simulink library "mobileRoboticsLib"  (R2018a)
settings: Solver=VariableStepAuto  StartTime=0.0  StopTime=10.0  RelTol=1e-3
undefined symbols (not defined in the file or in its folder): DiscIntNeverNeededParam, X, Y, Z
libraries: sm_lib x67, nesl_utility x25, $bdroot x11
(part 1 of 4)
settings Model: Creator=scastro  LastModifiedBy=scastro

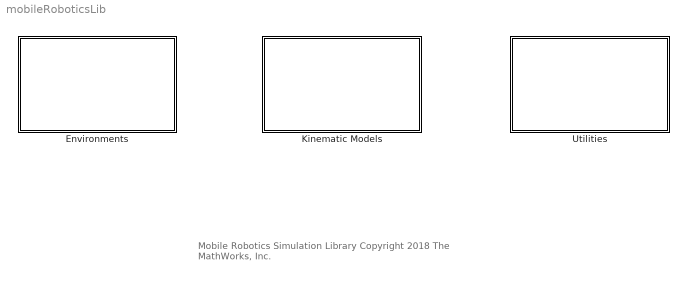
== system mobileRoboticsLib ==
  note: Mobile Robotics Simulation Library
      |
      | Copyright 2018 The MathWorks, Inc.
  Environments : Subsystem
      mask Display: image('environments.PNG');
  Kinematic Models : Subsystem
      mask Display: image('kinematics.PNG')
  Utilities : Subsystem
      mask Display: image('mrsUtils.PNG');

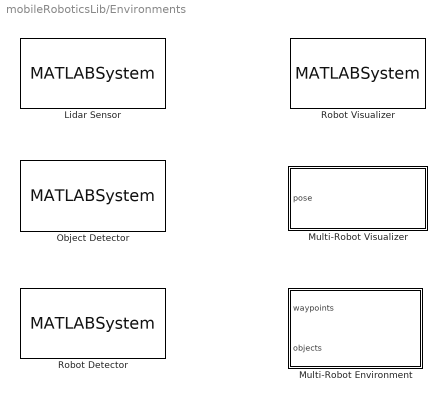
== system mobileRoboticsLib/Environments ==
  Lidar Sensor : MATLABSystem  System=LidarSensor  sensorOffset=[ 0, 0 ]  scanAngles=[ -pi/4, 0, pi/4 ]  maxRange=5  isMultiRobot=off  robotIdx=1
      mask Type: LidarSensor
      mask Display:
      | disp(['Lidar' char(10) 'Sensor']);
      | port_label('input',1,'pose');
      | port_label('output',1,'ranges');
  Multi-Robot Environment : Subsystem  InitFcn=|  TreatAsAtomicUnit=on  mask(Multi-Robot Environment){numRobots=3, mapName=, showWaypoints=on, showObjects=on, showRobotIds=on, plotSensorLines=on}
      | global slMultiRobotEnv;
      | numRobots = str2num(get_param(gcb,'numRobots'));
      | slMultiRobotEnv = MultiRobotEnv(numRobots);
      | slMultiRobotEnv.hasWaypoints = true;
      mask prompts: numRobots "Number of Robots"; mapName "Map Name"; showWaypoints "Accept Waypoints"; showObjects "Accept Objects"; showRobotIds "Show Robot IDs"; plotSensorLines "Plot Sensor Lines"
      mask help:
      | Displays map, waypoint, and object data for a multi-robot simulation.
      |
      | Use "Multi-Robot Visualizer" blocks to display individual robots in this environment.
      mask init:
      | % Configure waypoints port
      | hasWaypointPort = isempty(find_system(gcb,'FollowLinks','on','LookUnderMasks','on','BlockType','Inport','Name','waypoints'));
      | if ~showWaypoints & ~hasWaypointPort
      |     replace_block(gcb,'FollowLinks','on','Name','waypoints','built-in/Ground','noprompt');
      |     hasWaypointPort = false;
      | elseif showWaypoints & hasWaypointPort
      |     replace_block(gcb,'FollowLinks','on','Name','waypoints','built-in/Inport','noprompt'); 
      |     hasWaypointPort = true;
      | end
      | 
      | % Configure objects port
      | hasObjectPort = isempty(find_system(gcb,'FollowLinks','on','LookUnderMasks','on','BlockType','Inport','Name','objects'));
      | if ~showObjects & ~hasObjectPort
      |     replace_block(gcb,'FollowLinks','on','Name','objects','built-in/Ground','noprompt');
      |     hasObjectPort = false;
      | elseif showObjects & hasObjectPort
      |     replace_block(gcb,'FollowLinks','on','Name','objects','built-in/Inport','noprompt');  
      |     hasObjectPort = true;
      | end
      | 
      | % Ensure the waypoints and objects ports are organized correctly
      | if strcmp(get_param([gcb '/waypoints'],'BlockType'),'Inport')
      |     set_param([gcb '/waypoints'],'Port','1');
      | end
      | 
      | 
      | global slMultiRobotEnv
      | if isa(slMultiRobotEnv,'MultiRobotEnv')
      |     release(slMultiRobotEnv) 
      |     slMultiRobotEnv.numRobots = numRobots;
      |     slMultiRobotEnv.mapName = mapName;
      |     slMultiRobotEnv.plotSensorLines = plotSensorLines;
      |     slMultiRobotEnv.showRobotIds = showRobotIds;
      | 
      |     % Show the visualizer
      |     setupVisualization(slMultiRobotEnv);
      | end
      mask Help: web('matlab: edit mrsDocMultiRobotEnv')
      mask Display: fprintf('Multi-Robot\nEnvironment')
  Multi-Robot Visualizer : Subsystem  mask(Multi-Robot Visualizer){idx=1, radius=0, showTraj=on, hasLidar=off, sensorOffset=[0,0], scanAngles=[-pi/4, 0, pi/4], hasObjDetector=off, objDetectorOffset=[0,0], objDetectorAngle=0, objDetectorFOV=pi/3, objDetectorMaxRange=5}
      mask prompts: idx "Robot Index"; radius "Robot Radius [m]"; showTraj "Show Trajectory"; hasLidar "Accept Lidar"; sensorOffset "Lidar sensor offset (x,y) [m]"; scanAngles "Scan angles [rad]"; hasObjDetector "Accept Object Detector"; objDetectorOffset "Object detector offset (x,y) [m]"; objDetectorAngle "Object detector angle [rad]"; objDetectorFOV "Sensor field of view [rad]"; objDetectorMaxRange "Maximum range [m]"
      mask help:
      | Supply the pose and (optionally) lidar ranges for a single robot in a multi-robot setup.
      |
      | These blocks require a "Multi-Robot Environment" block to exist in the model.
      mask init:
      | % Configure ranges port
      | if ~hasLidar & ~isempty(find_system(gcb,'FollowLinks','on','LookUnderMasks','on','BlockType','Inport','Name','ranges'))
      |     replace_block(gcb,'FollowLinks','on','Name','ranges','built-in/Ground','noprompt');
      | elseif hasLidar & isempty(find_system(gcb,'FollowLinks','on','LookUnderMasks','on','BlockType','Inport','Name','ranges'))
      |     replace_block(gcb,'FollowLinks','on','Name','ranges','built-in/Inport','noprompt');  
      | end
      | 
      | global slMultiRobotEnv
      | if isa(slMultiRobotEnv,'MultiRobotEnv')
      |     release(slMultiRobotEnv)
      | 
      |     % Radius setting
      |     slMultiRobotEnv.robotRadius(idx) = radius;
      | 
      |     % Trajectory setting
      |     slMultiRobotEnv.showTrajectory(idx) = showTraj;
      | 
      |     % Lidar property setting
      |     slMultiRobotEnv.hasLidar(idx) = hasLidar;
      |     slMultiRobotEnv.scanAngles{idx} = scanAngles;
      |     slMultiRobotEnv.sensorOffset{idx} = sensorOffset;
      | 
      |     % Object detector property setting
      |     slMultiRobotEnv.hasObjDetector(idx) = hasObjDetector;
      |     slMultiRobotEnv.objDetectorOffset{idx} = objDetectorOffset;
      |     slMultiRobotEnv.objDetectorAngle(idx) = objDetectorAngle;
      |     slMultiRobotEnv.objDetectorFOV(idx) = objDetectorFOV;
      |     slMultiRobotEnv.objDetectorMaxRange(idx) = objDetectorMaxRange;
      | 
      | end
      mask Help: web('matlab: edit mrsDocMultiRobotEnv')
      mask Callback hasLidar:
      | mask = Simulink.Mask.get(gcb);
      | hasLidar = get_param(gcb,'hasLidar');
      | 
      | % Enable and disable parameters
      | indices = [find(strcmp({mask.Parameters.Name},'sensorOffset'));
      |            find(strcmp({mask.Parameters.Name},'scanAngles'))];
      | 
      | for idx = 1:numel(indices)
      |     mask.Parameters(indices(idx)).Visible = hasLidar;
      | end
      mask Callback hasObjDetector:
      | mask = Simulink.Mask.get(gcb);
      | hasObjDetector = get_param(gcb,'hasObjDetector');
      | 
      | indices = [find(strcmp({mask.Parameters.Name},'objDetectorOffset'));
      |            find(strcmp({mask.Parameters.Name},'objDetectorAngle'));
      |            find(strcmp({mask.Parameters.Name},'objDetectorFOV'));
      |            find(strcmp({mask.Parameters.Name},'objDetectorMaxRange'))];
      | 
      | for idx = 1:numel(indices)
      |     mask.Parameters(indices(idx)).Visible = hasObjDetector;
      | end
      mask Display:
      | idx = get_param(gcb,'idx');
      | fprintf(['Robot ' idx '\n Visualizer'])
  Object Detector : MATLABSystem  System=ObjectDetector  sensorOffset=[ 0, 0 ]  sensorAngle=0  fieldOfView=pi/3  maxRange=5  maxDetections=3  sampleTime=0.1
      mask Type: ObjectDetector
      mask Display:
      | disp(['Object' char(10) 'Detector']);
      | port_label('input',1,'pose');
      | port_label('input',2,'objects');
      | port_label('output',1,'detections');
  Robot Detector : MATLABSystem  System=RobotDetector  robotIdx=1  sensorOffset=[ 0, 0 ]  sensorAngle=0  fieldOfView=pi/3  maxRange=5  maxDetections=3  sampleTime=0.1
      mask Type: RobotDetector
      mask Display:
      | disp(['Robot 1' char(10) 'Detector']);
      | port_label('output',1,'detections');
  Robot Visualizer : MATLABSystem  System=Visualizer2D  robotRadius=0  showTrajectory=on  hasWaypoints=off  hasLidar=off  sensorOffset=[ 0, 0 ]  scanAngles=[ -pi/4, 0, pi/4 ]  hasObjDetector=off  objDetectorOffset=[ 0, 0 ]  objDetectorAngle=0  objDetectorFOV=pi/4  objDetectorMaxRange=5  objectColors=[ 1, 0, 0; 0, 1, 0; 0, 0, 1 ]
      mask Type: Visualizer2D
      mask Display:
      | disp(['Robot' char(10) 'Visualizer']);
      | port_label('input',1,'pose');

== system mobileRoboticsLib/Kinematic Models ==
  Differential Drive : Subsystem
      mask Display: image('diffDriveIcon.PNG')
  Four-Wheel Mecanum : Subsystem
      mask Display: image('mecanumIcon.PNG')
  Four-Wheel Steering : Subsystem
      mask Display: image('fourWheelSteerIcon.PNG')
  Generic Omniwheel : Subsystem
      mask Display: image('genericOmniIcon.png')
  Triple Omniwheel : Subsystem
      mask Display: image('tripleOmniIcon.PNG')

== system mobileRoboticsLib/Utilities ==
  Body to World Velocity : Subsystem  mask(Body to World Velocity){}
      mask help:
      | Converts a 2D velocity input [vx;vy;w] from body (vehicle) coordinates to world (global) coordinates.
      |
      | vx = Linear velocity in x-direction (longitudinal)
      | vy = Linear velocity in y-direction (lateral)
      | w = Angular velocity (about z-axis)
  Generic Vehicle Simulation : Subsystem  mask(Generic Vehicle Simulation){initX=2, initY=3, initAngle=0, Ts=0.05}
      mask prompts: initX "Initial X Position [m]"; initY "Initial Y Position [m]"; initAngle "Initial Angle (theta) [rad]"; Ts "Sample Time"
      mask help:
      | Simulates the kinematics of a generic vehicle, from a specified initial pose.
      |
      | Input: Body velocities [vx; vy; w], in m/s, m/s, and rad/s
      |
      | Output: Pose [x; y; theta], in m, m, and rad
      |
      | Set the Sample Time parameter to 0 for continuous-time simulation, or a positive number for discrete-time simulation.
      mask init:
      | blk = [gcb '/Velocity Integrator'];
      | if Ts > 0
      |     set_param(blk,'OverrideUsingVariant','mode==2');  
      | else
      |     set_param(blk,'OverrideUsingVariant','mode==1');  
      | end
  World to Body Velocity : Subsystem  mask(World to Body Velocity){}
      mask help:
      | Converts a 2D velocity input [vx;vy;w] from world (global) coordinates to body (vehicle) coordinates.
      |
      | vx = Linear velocity in x-direction (longitudinal)
      | vy = Linear velocity in y-direction (lateral)
      | w = Angular velocity (about z-axis)

== system mobileRoboticsLib/Environments/Multi-Robot Environment ==
  waypoints : Inport
  objects : Inport  Port=2
  MATLAB Function : MATLAB Function  TreatAsAtomicUnit=on
  wires:
  waypoints/1 -> MATLAB Function/1(wps)
  objects/1 -> MATLAB Function/2(objs)

== system mobileRoboticsLib/Environments/Multi-Robot Visualizer ==
  pose : Inport
  MATLAB Function : MATLAB Function  TreatAsAtomicUnit=on
  ranges : Ground
  wires:
  ranges/1 -> MATLAB Function/2(rngs)
  pose/1 -> MATLAB Function/1(pose)

== system mobileRoboticsLib/Kinematic Models/Differential Drive ==
  Differential Drive (Simscape Multibody Model) : Subsystem  mask(Differential Drive (Simscape Multibody Model)){wheelRadius=0.1, wheelBase=0.5, wheelThickness=0.025, chassisThickness=0.05, initX=0, initY=0, initAngle=0, timeConstant=0.05, wheelMass=0.1, chassisMass=1, wheelColor=[0.25 0.25 0.25], chassisColor=[0.8 0 0]}
      mask prompts: wheelRadius "Wheel Radius [m]"; wheelBase "Wheelbase [m]"; wheelThickness "Wheel Thickness [m]"; chassisThickness "Chassis Thickness [m]"; initX "Initial X Position [m]"; initY "Initial Y Position [m]"; initAngle "Initial Angle [rad]"; timeConstant "Motion Time Constant [s]"; wheelMass "Wheel Mass [kg]"; chassisMass "Chassis Mass [kg]"; wheelColor "Wheel Color"; chassisColor "Chassis Color"
      mask help:
      | Kinematics-only (motion actuated) Simscape Multibody Model of a differential drive vehicle.
      |
      | Inputs:
      | Left and right wheel speeds [wL; wR], in rad/s
      | Pose [x; y; theta], in m, m, and rad/s, respectively
      |
      | Connection Ports:
      | R: Reference frame at center of vehicle
      | G: Ground/world location
      mask Help: web('matlab:edit mrsDocDifferentialDrive')
      mask DialogControl KinContainer Prompt: Kinematics
      mask DialogControl DynamicsContainer Prompt: Dynamics
      mask DialogControl AppearanceContainer Prompt: Appearance
  Differential Drive Forward Kinematics : Subsystem  mask(Differential Drive Forward Kinematics){wheelRadius=0.1, wheelBase=0.5}
      mask prompts: wheelRadius "Wheel Radius [m]"; wheelBase "Wheelbase [m]"
      mask help:
      | Calculates the forward kinematics for a differential drive vehicle.
      |
      | Input: [wL; wR], the left and right wheel speeds (rad/s)
      |
      | Output: [v; w], the linear (m/s) and angular (rad/s) velocities of the vehicle
      mask Help: web('matlab:edit mrsDocDifferentialDrive')
  Differential Drive Inverse Kinematics : Subsystem  mask(Differential Drive Inverse Kinematics){wheelRadius=0.1, wheelBase=0.5}
      mask prompts: wheelRadius "Wheel Radius [m]"; wheelBase "Wheelbase [m]"
      mask help:
      | Calculates the forward kinematics for a differential drive vehicle.
      |
      | Input: [v; w], the linear (m/s) and angular (rad/s) velocities of the vehicle
      |
      | Output: [wL; wR], the left and right wheel speeds (rad/s)
      mask Help: web('matlab:edit mrsDocDifferentialDrive')
  Differential Drive Simulation : Subsystem  mask(Differential Drive Simulation){wheelRadius=0.1, wheelBase=0.5, initX=0, initY=0, initAngle=0, Ts=0.05}
      mask prompts: wheelRadius "Wheel Radius [m]"; wheelBase "Wheelbase [m]"; initX "Initial X Position [m]"; initY "Initial Y Position [m]"; initAngle "Initial Angle [rad]"; Ts "Sample Time"
      mask help:
      | Simulates the kinematics of a differential drive vehicle from a specified initial pose.
      |
      | Input: Left and right wheel speeds [wL; wR], in rad/s
      |
      | Output: Pose [x; y; theta], in m, m, and rad
      |
      | Set the Sample Time parameter to 0 for continuous-time simulation, or a positive number for discrete-time simulation.
      mask Help: web('matlab:edit mrsDocDifferentialDrive')

== system mobileRoboticsLib/Kinematic Models/Four-Wheel Mecanum ==
  Four-Wheel Mecanum (Simscape Multibody Model) : Subsystem  mask(Four-Wheel Mecanum (Simscape Multibody Model)){wheelRadius=0.1, wheelBase=0.4, wheelTrack=0.5, wheelThickness=0.025, chassisThickness=0.05, initX=0, initY=0, initAngle=0, timeConstant=0.05, wheelMass=0.1, chassisMass=1, wheelColor=[0.25 0.25 0.25], chassisColor=[0.8 0 0]}
      mask prompts: wheelRadius "Wheel Radius [m]"; wheelBase "Wheelbase [m]"; wheelTrack "Track [m]"; wheelThickness "Wheel Thickness [m]"; chassisThickness "Chassis Thickness [m]"; initX "Initial X Position [m]"; initY "Initial Y Position [m]"; initAngle "Initial Angle [rad]"; timeConstant "Motion Time Constant [s]"; wheelMass "Wheel Mass [kg]"; chassisMass "Chassis Mass [kg]"; wheelColor "Wheel Color"; chassisColor "Chassis Color"
      mask help:
      | Kinematics-only (motion actuated) Simscape Multibody Model of a four-wheeled vehicle with Mecanum wheels.
      |
      | Inputs:
      | Wheel speeds [w1; w2; w3; w4] (rad/s)
      | Pose [x; y; theta], in m, m, and rad/s, respectively
      |
      | Connection Ports:
      | R: Reference frame at center of vehicle
      | G: Ground/world location
      mask Help: web('matlab:edit mrsDocFourWheelMecanum')
      mask DialogControl KinContainer Prompt: Kinematics
      mask DialogControl DynamicsContainer Prompt: Dynamics
      mask DialogControl AppearanceContainer Prompt: Appearance
  Four-Wheel Mecanum Forward Kinematics : Subsystem  mask(Four-Wheel Mecanum Forward Kinematics){wheelRadius=0.1, wheelBase=0.4, wheelTrack=0.5}
      mask prompts: wheelRadius "Wheel Radius [m]"; wheelBase "Wheelbase [m]"; wheelTrack "Track [m]"
      mask help:
      | Calculates the forward kinematics for a four-wheeled vehicle with Mecanum wheels.
      |
      | Input: Wheel speeds [w1; w2; w3; w4] (rad/s)
      |
      | Output: Vehicle velocities [vx; vy; w] in body coordinates (m/s, m/s, and rad/s)
      mask Help: web('matlab:edit mrsDocFourWheelMecanum')
  Four-Wheel Mecanum Inverse Kinematics : Subsystem  mask(Four-Wheel Mecanum Inverse Kinematics){wheelRadius=0.1, wheelBase=0.4, wheelTrack=0.5}
      mask prompts: wheelRadius "Wheel Radius [m]"; wheelBase "Wheelbase [m]"; wheelTrack "Track [m]"
      mask help:
      | Calculates the inverse kinematics for a four-wheeled vehicle with Mecanum wheels.
      |
      | Input: Vehicle velocities [vx; vy; w] in body coordinates (m/s, m/s, and rad/s)
      |
      | Output: Wheel speeds [w1; w2; w3; w4] (rad/s)
      mask Help: web('matlab:edit mrsDocFourWheelMecanum')
  Four-Wheel Mecanum Simulation : Subsystem  mask(Four-Wheel Mecanum Simulation){wheelRadius=0.1, wheelBase=0.4, wheelTrack=0.5, initX=0, initY=0, initAngle=0, Ts=0.05}
      mask prompts: wheelRadius "Wheel Radius [m]"; wheelBase "Wheelbase [m]"; wheelTrack "Track [m]"; initX "Initial X Position [m]"; initY "Initial Y Position [m]"; initAngle "Initial Angle [rad]"; Ts "Sample Time"
      mask help:
      | Simulates the kinematics of a four-wheeled vehicle with Mecanum wheels, from a specified initial pose.
      |
      | Input: Wheel speeds [w1; w2; w3; w4] (rad/s)
      |
      | Output: Pose [x; y; theta], in m, m, and rad
      |
      | Set the Sample Time parameter to 0 for continuous-time simulation, or a positive number for discrete-time simulation.
      mask Help: web('matlab:edit mrsDocFourWheelMecanum')

== system mobileRoboticsLib/Kinematic Models/Four-Wheel Steering ==
  Four-Wheel Steering (Simscape Multibody Model) : Subsystem  mask(Four-Wheel Steering (Simscape Multibody Model)){wheelRadius=0.1, wheelBase=0.3, frontLen=0.25, rearLen=0.25, wheelThickness=0.025, chassisThickness=0.05, initX=0, initY=0, initAngle=0, timeConstant=0.05, wheelMass=0.1, chassisMass=1, wheelColor=[0.25 0.25 0.25], chassisColor=[0.8 0 0]}
      mask prompts: wheelRadius "Wheel Radius [m]"; wheelBase "Wheelbase [m]"; frontLen "CG to Front Wheel Distance [m]"; rearLen "CG to Rear Wheel Distance [m]"; wheelThickness "Wheel Thickness [m]"; chassisThickness "Chassis Thickness [m]"; initX "Initial X Position [m]"; initY "Initial Y Position [m]"; initAngle "Initial Angle [rad]"; timeConstant "Motion Time Constant [s]"; wheelMass "Wheel Mass [kg]"; chassisMass "Chassis Mass [kg]"; wheelColor "Wheel Color"; chassisColor "Chassis Color"
      mask help:
      | Kinematics-only (motion actuated) Simscape Multibody Model of a four-wheeled vehicle with front and rear drive and steering.
      |
      | Input:
      | Wheel speeds [wf; wr] (rad/s)
      | Steer angles [phif; phir] (rad)
      | Pose [x; y; theta], in m, m, and rad/s, respectively
      |
      | Connection Ports:
      | R: Reference frame at center of vehicle
      | G: Ground/world location
      mask Help: web('matlab:edit mrsDocFourWheelSteer')
      mask DialogControl KinContainer Prompt: Kinematics
      mask DialogControl DynamicsContainer Prompt: Dynamics
      mask DialogControl AppearanceContainer Prompt: Appearance
  Four-Wheel Steering Forward Kinematics : Subsystem  mask(Four-Wheel Steering Forward Kinematics){wheelRadius=0.1, frontWheelDist=0.25, rearWheelDist=0.25}
      mask prompts: wheelRadius "Wheel Radius [m]"; frontWheelDist "CG to Front Wheel Distance [m]"; rearWheelDist "CG to Rear Wheel Distance [m]"
      mask help:
      | Calculates the forward kinematics for a four-wheeled vehicle with front and rear drive and steering.
      |
      | Input:
      | Wheel speeds [wf; wr] (rad/s)
      | Steer angles [phif; phir] (rad)
      |
      | Output: Vehicle velocities [vx; vy; w] in body coordinates (m/s, m/s, and rad/s)
      mask Help: web('matlab:edit mrsDocFourWheelSteer')
  Four-Wheel Steering Inverse Kinematics : Subsystem  mask(Four-Wheel Steering Inverse Kinematics){wheelRadius=0.1, frontWheelDist=0.25, rearWheelDist=0.25, ikMode=Front Steering}
      mask prompts: wheelRadius "Wheel Radius [m]"; frontWheelDist "CG to Front Wheel Distance [m]"; rearWheelDist "CG to Rear Wheel Distance [m]"; ikMode "Inverse Kinematics Mode"
      mask help:
      | Calculates the inverse kinematics for a four-wheeled vehicle with front and rear drive and steering.
      |
      | Input:
      | Vehicle velocities [vx; vy; w] in body coordinates (m/s, m/s, and rad/s)
      | In Front Steering and Zero Sideslip mode, the velocity inputs used are forward and angular speed [vx;w]
      | In Parallel Steering mode, the velocity inputs used are forward and lateral speed [vx;vy]
      |
      | Output:
      | Wheel speeds [wf; wr] (rad/s)
      | Steer angles [phif; phir] (rad)
      mask init:
      | blk = [gcb '/Inverse Kinematics'];
      | varStr = ['mode==' num2str(ikMode)];
      | set_param(blk,'OverrideUsingVariant',varStr);
      mask Help: web('matlab:edit mrsDocFourWheelSteer')
      mask TypeOptions ikMode: Front Steering | Parallel Steering | Zero Sideslip
      mask Display:
      | text(0.5,0.9,get_param(gcb,'ikMode'), ...
      |      'horizontalAlignment','center');
  Four-Wheel Steering Simulation : Subsystem  mask(Four-Wheel Steering Simulation){wheelRadius=0.1, frontWheelDist=0.25, rearWheelDist=0.25, initX=0, initY=0, initAngle=0, Ts=0.05}
      mask prompts: wheelRadius "Wheel Radius [m]"; frontWheelDist "CG to Front Wheel Distance [m]"; rearWheelDist "CG to Rear Wheel Distance [m]"; initX "Initial X Position [m]"; initY "Initial Y Position [m]"; initAngle "Initial Angle [rad]"; Ts "Sample Time"
      mask help:
      | Simulates the kinematics of a four-wheeled vehicle with front and rear drive and steering, from a specified initial pose.
      |
      | Input:
      | Wheel speeds [wf; wr] (rad/s)
      | Steer angles [phif; phir] (rad)
      |
      | Output: Pose [x; y; theta], in m, m, and rad
      |
      | Set the Sample Time parameter to 0 for continuous-time simulation, or a positive number for discrete-time simulation.
      mask Help: web('matlab:edit mrsDocFourWheelSteer')

== system mobileRoboticsLib/Kinematic Models/Generic Omniwheel ==
  Generic Omniwheel Forward Kinematics : Subsystem  mask(Generic Omniwheel Forward Kinematics){wheelRadius=0.1, wheelPositions=[1 1;-1 1;-1 -1;1 -1], wheelAngles=[0; pi/4; -pi/4; 0]}
      mask prompts: wheelRadius "Wheel Radius [m]"; wheelPositions "Wheel (X,Y) Positions [m]"; wheelAngles "Wheel Angles [rad]"
      mask help:
      | Calculates the forward kinematics for an N-wheeled vehicle with omniwheels.
      |
      | Input: Wheel speeds [w1; w2; ... ; wN] (rad/s)
      |
      | Output: Vehicle velocities [vx; vy; w] in body coordinates (m/s, m/s, and rad/s)
      mask Help: web('matlab:edit mrsDocGenericOmniwheel')
  "Generic Omniwheel Inverse Kinematics " : Subsystem  mask(Generic Omniwheel Inverse Kinematics){wheelRadius=0.1, wheelPositions=[1 1;-1 1;-1 -1;1 -1], wheelAngles=[0; pi/4; -pi/4; 0]}
      mask prompts: wheelRadius "Wheel Radius [m]"; wheelPositions "Wheel (X,Y) Positions [m]"; wheelAngles "Wheel Angles [rad]"
      mask help:
      | Calculates the inverse kinematics for an N-wheeled vehicle with omniwheels.
      |
      | Input: Vehicle velocities [vx; vy; w] in body coordinates (m/s, m/s, and rad/s)
      |
      | Output: Wheel speeds [w1; w2; ... ; wN] (rad/s)
      mask Help: web('matlab:edit mrsDocGenericOmniwheel')
  Generic Omniwheel Simulation : Subsystem  mask(Generic Omniwheel Simulation){wheelRadius=0.1, wheelPositions=[1 1;-1 1;-1 -1;1 -1], wheelAngles=[0; pi/4; -pi/4; 0], initX=0, initY=0, initAngle=0, Ts=0.05}
      mask prompts: wheelRadius "Wheel Radius [m]"; wheelPositions "Wheel (X,Y) Positions [m]"; wheelAngles "Wheel Angles [rad]"; initX "Initial X Position [m]"; initY "Initial Y Position [m]"; initAngle "Initial Angle [rad]"; Ts "Sample Time"
      mask help:
      | Simulates the kinematics of an N-wheeled vehicle with omniwheels, from a specified initial pose.
      |
      | Input: Wheel speeds [w1; w2; ... ; wN] (rad/s)
      |
      | Output: Pose [x; y; theta], in m, m, and rad
      |
      | Set the Sample Time parameter to 0 for continuous-time simulation, or a positive number for discrete-time simulation.
      mask Help: web('matlab:edit mrsDocGenericOmniwheel')

== system mobileRoboticsLib/Kinematic Models/Triple Omniwheel ==
  Triple Omniwheel (Simscape Multibody Model) : Subsystem  mask(Triple Omniwheel (Simscape Multibody Model)){wheelRadius=0.1, robotRadius=0.25, wheelAngles=[0,2*pi/3,-2*pi/3], wheelThickness=0.025, chassisThickness=0.05, initX=2, initY=3, initAngle=0, timeConstant=0.05, wheelMass=0.1, chassisMass=1, wheelColor=[0.25 0.25 0.25], chassisColor=[0.8 0 0]}
      mask prompts: wheelRadius "Wheel Radius [m]"; robotRadius "Robot Radius [m]"; wheelAngles "Wheel Angles [rad]"; wheelThickness "Wheel Thickness [m]"; chassisThickness "Chassis Thickness [m]"; initX "Initial X Position [m]"; initY "Initial Y Position [m]"; initAngle "Initial Angle [rad]"; timeConstant "Motion Time Constant [s]"; wheelMass "Wheel Mass [kg]"; chassisMass "Chassis Mass [kg]"; wheelColor "Wheel Color"; chassisColor "Chassis Color"
      mask help:
      | Kinematics-only (motion actuated) Simscape Multibody Model of a three-wheeled vehicle with omniwheels.
      |
      | Inputs:
      | Wheel speeds [w1; w2; w3] (rad/s)
      | Pose [x; y; theta], in m, m, and rad/s, respectively
      |
      | Connection Ports:
      | R: Reference frame at center of vehicle
      | G: Ground/world location
      mask Help: web('matlab:edit mrsDocTripleOmniwheel')
      mask DialogControl KinContainer Prompt: Kinematics
      mask DialogControl DynamicsContainer Prompt: Dynamics
      mask DialogControl AppearanceContainer Prompt: Appearance
  Triple Omniwheel Forward Kinematics : Subsystem  mask(Triple Omniwheel Forward Kinematics){wheelRadius=0.1, robotRadius=0.25, wheelAngles=[0,2*pi/3,-2*pi/3]}
      mask prompts: wheelRadius "Wheel Radius [m]"; robotRadius "Robot Radius [m]"; wheelAngles "Wheel Angles [rad]"
      mask help:
      | Calculates the forward kinematics for a three-wheeled vehicle with omniwheels.
      |
      | Input: Wheel speeds [w1; w2; w3] (rad/s)
      |
      | Output: Vehicle velocities [vx; vy; w] in body coordinates (m/s, m/s, and rad/s)
      mask Help: web('matlab:edit mrsDocTripleOmniwheel')
  "Triple Omniwheel Inverse Kinematics " : Subsystem  mask(Triple Omniwheel Inverse Kinematics){wheelRadius=0.1, robotRadius=0.25, wheelAngles=[0,2*pi/3,-2*pi/3]}
      mask prompts: wheelRadius "Wheel Radius [m]"; robotRadius "Robot Radius [m]"; wheelAngles "Wheel Angles [rad]"
      mask help:
      | Calculates the inverse kinematics for a three-wheeled vehicle with omniwheels.
      |
      | Input: Vehicle velocities [vx; vy; w] in body coordinates (m/s, m/s, and rad/s)
      |
      | Output: Wheel speeds [w1; w2; w3] (rad/s)
      mask Help: web('matlab:edit mrsDocTripleOmniwheel')
  Triple Omniwheel Simulation : Subsystem  mask(Triple Omniwheel Simulation){wheelRadius=0.1, robotRadius=0.25, wheelAngles=[0,2*pi/3,-2*pi/3], initX=0, initY=0, initAngle=0, Ts=0.05}
      mask prompts: wheelRadius "Wheel Radius [m]"; robotRadius "Robot Radius [m]"; wheelAngles "Wheel Angles [rad]"; initX "Initial X Position [m]"; initY "Initial Y Position [m]"; initAngle "Initial Angle [rad]"; Ts "Sample Time"
      mask help:
      | Simulates the kinematics of a three-wheeled vehicle with omniwheels, from a specified initial pose.
      |
      | Input: Wheel speeds [w1; w2; w3] (rad/s)
      |
      | Output: Pose [x; y; theta], in m, m, and rad
      |
      | Set the Sample Time parameter to 0 for continuous-time simulation, or a positive number for discrete-time simulation.
      mask Help: web('matlab:edit mrsDocTripleOmniwheel')

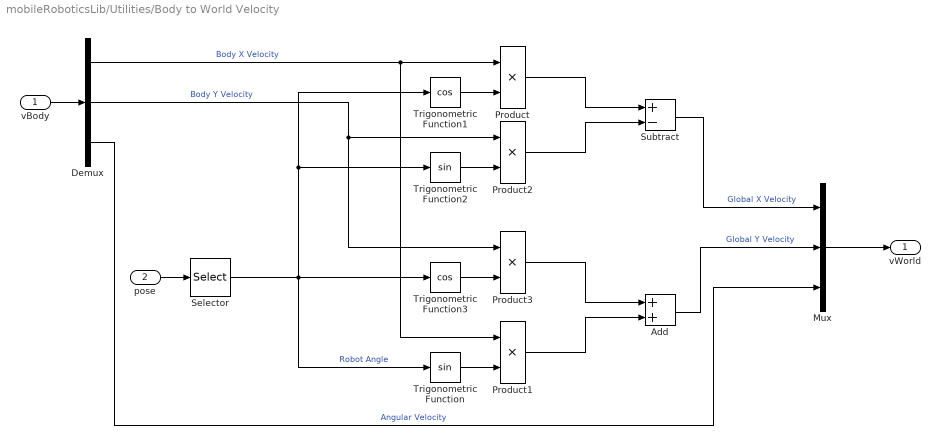
== system mobileRoboticsLib/Utilities/Body to World Velocity ==
  vBody : Inport
  pose : Inport  Port=2
  Add : Sum
  Demux : Demux  Outputs=3
  Mux : Mux  Inputs=3
  Product{,1..3} (4 alike) : Product
  Selector : Selector  InputPortWidth=3  IndexOptions=Index vector (dialog)  Indices=3  OutputSizes=1
  Subtract : Sum  Inputs=+-
  Trigonometric Function : Trigonometry
  Trigonometric Function1 : Trigonometry  Operator=cos
  Trigonometric Function2 : Trigonometry
  Trigonometric Function3 : Trigonometry  Operator=cos
  vWorld : Outport
  wires:
  pose/1 -> Selector/1
  Add/1 -> Mux/2  "Global Y Velocity"
  Product3/1 -> Add/1
  Trigonometric Function3/1 -> Product3/2
  Product2/1 -> Subtract/2
  Demux/2 -> Product2/1, Product3/1  "Body Y Velocity"
  Trigonometric Function2/1 -> Product2/2
  Subtract/1 -> Mux/1  "Global X Velocity"
  Selector/1 -> Trigonometric Function/1, Trigonometric Function1/1, Trigonometric Function2/1, Trigonometric Function3/1  "Robot Angle"
  Demux/1 -> Product/1, Product1/1  "Body X Velocity"
  Trigonometric Function1/1 -> Product/2
  Product/1 -> Subtract/1
  Product1/1 -> Add/2
  Trigonometric Function/1 -> Product1/2
  vBody/1 -> Demux/1
  Mux/1 -> vWorld/1
  Demux/3 -> Mux/3  "Angular Velocity"

== system mobileRoboticsLib/Utilities/Generic Vehicle Simulation ==
  bodySpd : Inport
  Body to Cartesian Velocity : $bdroot/Utilities/Body to World Velocity
  Demux1 : Demux  Outputs=3
  Mux : Mux  Inputs=3
  Velocity Integrator : Subsystem  Variant=on  VariantControl=Variant1  OverrideUsingVariant=mode==2
  pose : Outport
  wires:
  bodySpd/1 -> Body to Cartesian Velocity/1
  Demux1/3 -> Velocity Integrator/3("w ")
  Demux1/2 -> Velocity Integrator/2("vy ")
  Demux1/1 -> Velocity Integrator/1("vx ")
  Body to Cartesian Velocity/1 -> Demux1/1
  Mux/1 -> pose/1, Body to Cartesian Velocity/2
  Velocity Integrator/1(" x") -> Mux/1
  Velocity Integrator/2(" y") -> Mux/2
  Velocity Integrator/3(" theta") -> Mux/3

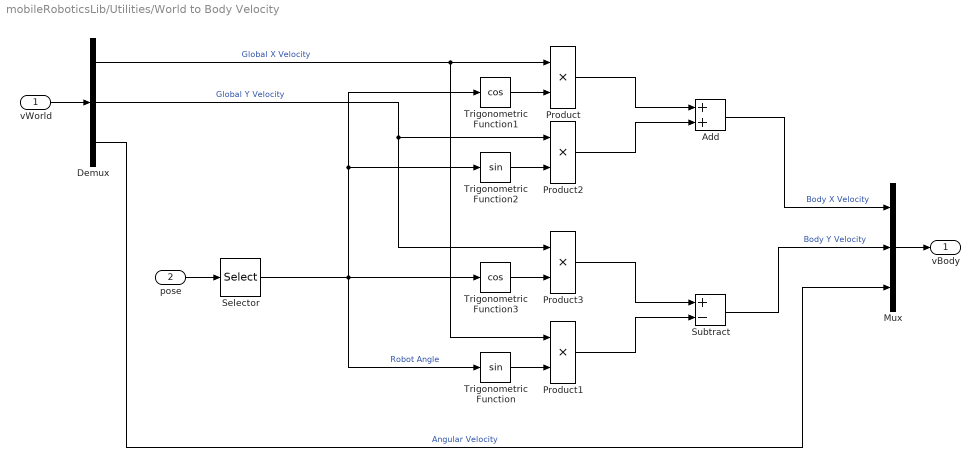
== system mobileRoboticsLib/Utilities/World to Body Velocity ==
  vWorld : Inport
  pose : Inport  Port=2
  Add : Sum
  Demux : Demux  Outputs=3
  Mux : Mux  Inputs=3
  Product{,1..3} (4 alike) : Product
  Selector : Selector  InputPortWidth=3  IndexOptions=Index vector (dialog)  Indices=3  OutputSizes=1
  Subtract : Sum  Inputs=+-
  Trigonometric Function : Trigonometry
  Trigonometric Function1 : Trigonometry  Operator=cos
  Trigonometric Function2 : Trigonometry
  Trigonometric Function3 : Trigonometry  Operator=cos
  vBody : Outport
  wires:
  Trigonometric Function/1 -> Product1/2
  Product1/1 -> Subtract/2
  Product/1 -> Add/1
  Trigonometric Function1/1 -> Product/2
  Demux/1 -> Product/1, Product1/1  "Global X Velocity"
  Selector/1 -> Trigonometric Function/1, Trigonometric Function3/1, Trigonometric Function2/1, Trigonometric Function1/1  "Robot Angle"
  Add/1 -> Mux/1  "Body X Velocity"
  Trigonometric Function2/1 -> Product2/2
  Demux/2 -> Product3/1, Product2/1  "Global Y Velocity"
  Product2/1 -> Add/2
  Trigonometric Function3/1 -> Product3/2
  Product3/1 -> Subtract/1
  Subtract/1 -> Mux/2  "Body Y Velocity"
  vWorld/1 -> Demux/1
  Demux/3 -> Mux/3  "Angular Velocity"
  Mux/1 -> vBody/1
  pose/1 -> Selector/1

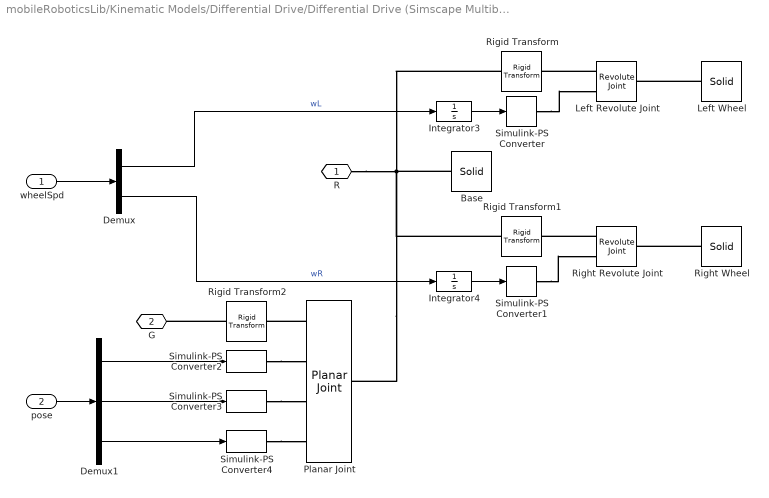
== system mobileRoboticsLib/Kinematic Models/Differential Drive/Differential Drive (Simscape Multibody Model) ==
  wheelSpd : Inport
  pose : Inport  Port=2
  Base : sm_lib/Body Elements/Solid  InertiaType=CalculateFromGeometry  Mass=chassisMass  MassUnits=kg  CenterOfMass=[0 0 0]  CenterOfMassUnits=m  MomentsOfInertia=[1 1 1]  MomentsOfInertiaUnits=kg*m^2  ProductsOfInertia=[1 1 1]  ProductsOfInertiaUnits=kg*m^2  DensityBased=off  Density=chassisMass  DensityUnits=kg/m^3  DoExposeReferenceFrame=on  SerializedFrames=<Frames/>  GraphicType=FromGeometry  MarkerShape=Sphere  MarkerSize=10  GraphicVisPropType=SimpleVisualProperties  GraphicDiffuseColor=chassisColor  GraphicSpecularColor=[0.5 0.5 0.5 1.0]  GraphicAmbientColor=[0.15 0.15 0.15 1.0]  GraphicEmissiveColor=[0.0 0.0 0.0 1.0]  GraphicShininess=75  GraphicOpacity=1.0  GeometryShape=Cylinder  RectangleSize=[1 1]  RectangleSizeUnits=m  BrickDimensions=[1 1 1]  BrickDimensionUnits=m  CylinderRadius=(wheelBase-wheelThickness)/2  CylinderRadiusUnits=m  CylinderLength=chassisThickness  CylinderLengthUnits=m  SphereRadius=1  SphereRadiusUnits=m  EllipsoidRadii=[1 1 1]  EllipsoidRadiiUnits=m  ExtrusionCrossSection=[1 1; -1 1; -1 -1; 1 -1]  ExtrusionCrossSectionUnits=m  ExtrusionLength=1  ExtrusionLengthUnits=m  PolygonNumSides=3  PolygonOuterRadius=1  PolygonOuterRadiusUnits=m  ExtGeomFileType=STEP  ExtGeomFileUnits=m  RevolutionCrossSection=[1 1; 1 -1; 2 -1; 2 1]  RevolutionCrossSectionUnits=m  RevolutionExtent=Full  RevolutionAngle=180  RevolutionAngleUnits=deg
  Demux : Demux  Outputs=2
  Demux1 : Demux  Outputs=3
  Integrator3 : Integrator
  Integrator4 : Integrator
  Left Revolute Joint : sm_lib/Joints/Revolute Joint  SenseConstraintForce=off  SenseConstraintForceX=off  SenseConstraintForceY=off  SenseConstraintForceZ=off  SenseConstraintTorque=off  SenseConstraintTorqueX=off  SenseConstraintTorqueY=off  SenseConstraintTorqueZ=off  SenseTotalForce=off  SenseTotalForceX=off  SenseTotalForceY=off  SenseTotalForceZ=off  SenseTotalTorque=off  SenseTotalTorqueX=off  SenseTotalTorqueY=off  SenseTotalTorqueZ=off  CompositeWrenchDir=FollowerOnBase  CompositeWrenchFrame=BaseFrame  EquilibriumPosition=0  EquilibriumPositionUnits=deg  SpringStiffness=0  SpringStiffnessUnits=N*m/deg  DampingCoefficient=0  DampingCoefficientUnits=N*m/(deg/s)  TorqueActuationMode=ComputedTorque  MotionActuationMode=InputMotion  SensePosition=off  SenseVelocity=off  SenseAcceleration=off  SenseTorqueForce=off  PositionTargetSpecify=off  PositionTargetPriority=High  PositionTargetValue=0  PositionTargetValueUnits=deg  VelocityTargetSpecify=off  VelocityTargetPriority=High  VelocityTargetValue=0  VelocityTargetValueUnits=deg/s
  Left Wheel : sm_lib/Body Elements/Solid  InertiaType=CalculateFromGeometry  Mass=wheelMass  MassUnits=kg  CenterOfMass=[0 0 0]  CenterOfMassUnits=m  MomentsOfInertia=[1 1 1]  MomentsOfInertiaUnits=kg*m^2  ProductsOfInertia=[1 1 1]  ProductsOfInertiaUnits=kg*m^2  DensityBased=off  Density=1000  DensityUnits=kg/m^3  DoExposeReferenceFrame=on  SerializedFrames=<Frames/>  GraphicType=FromGeometry  MarkerShape=Sphere  MarkerSize=10  GraphicVisPropType=SimpleVisualProperties  GraphicDiffuseColor=wheelColor  GraphicSpecularColor=[0.5 0.5 0.5 1.0]  GraphicAmbientColor=[0.15 0.15 0.15 1.0]  GraphicEmissiveColor=[0.0 0.0 0.0 1.0]  GraphicShininess=75  GraphicOpacity=1.0  GeometryShape=Cylinder  RectangleSize=[1 1]  RectangleSizeUnits=m  BrickDimensions=[1 1 1]  BrickDimensionUnits=m  CylinderRadius=wheelRadius  CylinderRadiusUnits=m  CylinderLength=wheelThickness  CylinderLengthUnits=m  SphereRadius=1  SphereRadiusUnits=m  EllipsoidRadii=[1 1 1]  EllipsoidRadiiUnits=m  ExtrusionCrossSection=[1 1; -1 1; -1 -1; 1 -1]  ExtrusionCrossSectionUnits=m  ExtrusionLength=1  ExtrusionLengthUnits=m  PolygonNumSides=3  PolygonOuterRadius=1  PolygonOuterRadiusUnits=m  ExtGeomFileType=STEP  ExtGeomFileUnits=m  RevolutionCrossSection=[1 1; 1 -1; 2 -1; 2 1]  RevolutionCrossSectionUnits=m  RevolutionExtent=Full  RevolutionAngle=180  RevolutionAngleUnits=deg
  Planar Joint : sm_lib/Joints/Planar Joint  SenseConstraintForce=off  SenseConstraintForceX=off  SenseConstraintForceY=off  SenseConstraintForceZ=off  SenseConstraintTorque=off  SenseConstraintTorqueX=off  SenseConstraintTorqueY=off  SenseConstraintTorqueZ=off  SenseTotalForce=off  SenseTotalForceX=off  SenseTotalForceY=off  SenseTotalForceZ=off  SenseTotalTorque=off  SenseTotalTorqueX=off  SenseTotalTorqueY=off  SenseTotalTorqueZ=off  CompositeWrenchDir=FollowerOnBase  CompositeWrenchFrame=BaseFrame  PxEquilibriumPosition=0  PxEquilibriumPositionUnits=m  PxSpringStiffness=0  PxSpringStiffnessUnits=N/m  PxDampingCoefficient=0  PxDampingCoefficientUnits=N/(m/s)  PxTorqueActuationMode=ComputedTorque  PxMotionActuationMode=InputMotion  PxSensePosition=off  PxSenseVelocity=off  PxSenseAcceleration=off  PxSenseTorqueForce=off  PxPositionTargetSpecify=on  PxPositionTargetPriority=High  PxPositionTargetValue=initX  PxPositionTargetValueUnits=m  PxVelocityTargetSpecify=off  PxVelocityTargetPriority=High  PxVelocityTargetValue=0  PxVelocityTargetValueUnits=m/s  PyEquilibriumPosition=0  PyEquilibriumPositionUnits=m  PySpringStiffness=0  PySpringStiffnessUnits=N/m  PyDampingCoefficient=0  PyDampingCoefficientUnits=N/(m/s)  PyTorqueActuationMode=ComputedTorque  PyMotionActuationMode=InputMotion  PySensePosition=off  PySenseVelocity=off  PySenseAcceleration=off  PySenseTorqueForce=off  PyPositionTargetSpecify=on  PyPositionTargetPriority=High  PyPositionTargetValue=initY  PyPositionTargetValueUnits=m  PyVelocityTargetSpecify=off  PyVelocityTargetPriority=High  PyVelocityTargetValue=0  PyVelocityTargetValueUnits=m/s  RzEquilibriumPosition=0  RzEquilibriumPositionUnits=deg  RzSpringStiffness=0  RzSpringStiffnessUnits=N*m/deg  RzDampingCoefficient=0  RzDampingCoefficientUnits=N*m/(deg/s)  RzTorqueActuationMode=ComputedTorque  RzMotionActuationMode=InputMotion  RzSensePosition=off  RzSenseVelocity=off  RzSenseAcceleration=off  RzSenseTorqueForce=off  RzPositionTargetSpecify=on  RzPositionTargetPriority=High  RzPositionTargetValue=initAngle  RzPositionTargetValueUnits=rad  RzVelocityTargetSpecify=off  RzVelocityTargetPriority=High  RzVelocityTargetValue=0  RzVelocityTargetValueUnits=deg/s
  Right Revolute Joint : sm_lib/Joints/Revolute Joint  SenseConstraintForce=off  SenseConstraintForceX=off  SenseConstraintForceY=off  SenseConstraintForceZ=off  SenseConstraintTorque=off  SenseConstraintTorqueX=off  SenseConstraintTorqueY=off  SenseConstraintTorqueZ=off  SenseTotalForce=off  SenseTotalForceX=off  SenseTotalForceY=off  SenseTotalForceZ=off  SenseTotalTorque=off  SenseTotalTorqueX=off  SenseTotalTorqueY=off  SenseTotalTorqueZ=off  CompositeWrenchDir=FollowerOnBase  CompositeWrenchFrame=BaseFrame  EquilibriumPosition=0  EquilibriumPositionUnits=deg  SpringStiffness=0  SpringStiffnessUnits=N*m/deg  DampingCoefficient=0  DampingCoefficientUnits=N*m/(deg/s)  TorqueActuationMode=ComputedTorque  MotionActuationMode=InputMotion  SensePosition=off  SenseVelocity=off  SenseAcceleration=off  SenseTorqueForce=off  PositionTargetSpecify=off  PositionTargetPriority=High  PositionTargetValue=0  PositionTargetValueUnits=deg  VelocityTargetSpecify=off  VelocityTargetPriority=High  VelocityTargetValue=0  VelocityTargetValueUnits=deg/s
  Right Wheel : sm_lib/Body Elements/Solid  InertiaType=CalculateFromGeometry  Mass=wheelMass  MassUnits=kg  CenterOfMass=[0 0 0]  CenterOfMassUnits=m  MomentsOfInertia=[1 1 1]  MomentsOfInertiaUnits=kg*m^2  ProductsOfInertia=[1 1 1]  ProductsOfInertiaUnits=kg*m^2  DensityBased=off  Density=1000  DensityUnits=kg/m^3  DoExposeReferenceFrame=on  SerializedFrames=<Frames/>  GraphicType=FromGeometry  MarkerShape=Sphere  MarkerSize=10  GraphicVisPropType=SimpleVisualProperties  GraphicDiffuseColor=wheelColor  GraphicSpecularColor=[0.5 0.5 0.5 1.0]  GraphicAmbientColor=[0.15 0.15 0.15 1.0]  GraphicEmissiveColor=[0.0 0.0 0.0 1.0]  GraphicShininess=75  GraphicOpacity=1.0  GeometryShape=Cylinder  RectangleSize=[1 1]  RectangleSizeUnits=m  BrickDimensions=[1 1 1]  BrickDimensionUnits=m  CylinderRadius=wheelRadius  CylinderRadiusUnits=m  CylinderLength=wheelThickness  CylinderLengthUnits=m  SphereRadius=1  SphereRadiusUnits=m  EllipsoidRadii=[1 1 1]  EllipsoidRadiiUnits=m  ExtrusionCrossSection=[1 1; -1 1; -1 -1; 1 -1]  ExtrusionCrossSectionUnits=m  ExtrusionLength=1  ExtrusionLengthUnits=m  PolygonNumSides=3  PolygonOuterRadius=1  PolygonOuterRadiusUnits=m  ExtGeomFileType=STEP  ExtGeomFileUnits=m  RevolutionCrossSection=[1 1; 1 -1; 2 -1; 2 1]  RevolutionCrossSectionUnits=m  RevolutionExtent=Full  RevolutionAngle=180  RevolutionAngleUnits=deg
  Rigid Transform : sm_lib/Frames and Transforms/Rigid Transform  TranslationMethod=StandardAxis  TranslationStandardOffset=wheelBase/2  TranslationLengthUnit=m  TranslationStandardAxis=+Y  TranslationCartesianOffset=[0 0 0]  TranslationROffset=0  TranslationROffsetUnits=m  TranslationZOffset=0  TranslationZOffsetUnits=m  TranslationThetaOffset=0  TranslationThetaOffsetUnits=deg  RotationMethod=AlignedAxes  RotationAngleUnits=deg  RotationStandardAxis=+Z  RotationAngle=0.0  RotationArbitraryAxis=[0 0 1]  FollAlignAxisA=+Z  BaseAlignAxisA=+Y  FollAlignAxisB=+X  BaseAlignAxisB=+X  RotationSequenceAxes=FollowerAxes  RotationSequence=XYX  RotationSequenceAngles=[0 0 0]  RotationSequenceAnglesUnits=deg  RotationMatrix=[1 0 0; 0 1 0; 0 0 1]
  Rigid Transform1 : sm_lib/Frames and Transforms/Rigid Transform  TranslationMethod=StandardAxis  TranslationStandardOffset=wheelBase/2  TranslationLengthUnit=m  TranslationStandardAxis=-Y  TranslationCartesianOffset=[0 0 0]  TranslationROffset=0  TranslationROffsetUnits=m  TranslationZOffset=0  TranslationZOffsetUnits=m  TranslationThetaOffset=0  TranslationThetaOffsetUnits=deg  RotationMethod=AlignedAxes  RotationAngleUnits=deg  RotationStandardAxis=+Z  RotationAngle=0.0  RotationArbitraryAxis=[0 0 1]  FollAlignAxisA=+Z  BaseAlignAxisA=+Y  FollAlignAxisB=+X  BaseAlignAxisB=+X  RotationSequenceAxes=FollowerAxes  RotationSequence=XYX  RotationSequenceAngles=[0 0 0]  RotationSequenceAnglesUnits=deg  RotationMatrix=[1 0 0; 0 1 0; 0 0 1]
  Rigid Transform2 : sm_lib/Frames and Transforms/Rigid Transform  TranslationMethod=StandardAxis  TranslationStandardOffset=wheelRadius  TranslationLengthUnit=m  TranslationStandardAxis=+Z  TranslationCartesianOffset=[0 0 0]  TranslationROffset=0  TranslationROffsetUnits=m  TranslationZOffset=0  TranslationZOffsetUnits=m  TranslationThetaOffset=0  TranslationThetaOffsetUnits=deg  RotationMethod=None  RotationAngleUnits=deg  RotationStandardAxis=+Z  RotationAngle=0.0  RotationArbitraryAxis=[0 0 1]  FollAlignAxisA=+Z  BaseAlignAxisA=+Y  FollAlignAxisB=+X  BaseAlignAxisB=+X  RotationSequenceAxes=FollowerAxes  RotationSequence=XYX  RotationSequenceAngles=[0 0 0]  RotationSequenceAnglesUnits=deg  RotationMatrix=[1 0 0; 0 1 0; 0 0 1]
  Simulink-PS Converter{,2..4} (4 alike) : nesl_utility/Simulink-PS Converter  PhysicalDomain=network_engine_domain  SubClassName=ps_input  LeftPortType=input  RightPortType=output  PseudoPeriodic=off  Frequencies=[]  NoiseDistribution=none  NoiseParameters=[]  Unit=1  AffineConversion=off  FilteringAndDerivatives=filter  SimscapeFilterOrder=2  InputFilterTimeConstant=timeConstant  UdotUserProvided=0
  Simulink-PS Converter1 : nesl_utility/Simulink-PS Converter  PhysicalDomain=network_engine_domain  SubClassName=ps_input  LeftPortType=input  RightPortType=output  PseudoPeriodic=off  Frequencies=[]  NoiseDistribution=none  NoiseParameters=[]  Unit=1  AffineConversion=off  FilteringAndDerivatives=filter  SimscapeFilterOrder=2  InputFilterTimeConstant=timeConstant  UdotUserProvided=2
  R : PMIOPort  Side=Right
  G : PMIOPort  Port=2  Side=Right
  wires:
  Integrator4/1 -> Simulink-PS Converter1/1
  Integrator3/1 -> Simulink-PS Converter/1
  Demux/2 -> Integrator4/1  "wR"
  Demux/1 -> Integrator3/1  "wL"
  wheelSpd/1 -> Demux/1
  pose/1 -> Demux1/1
  Demux1/1 -> Simulink-PS Converter2/1
  Demux1/2 -> Simulink-PS Converter3/1
  Demux1/3 -> Simulink-PS Converter4/1
  connections:
  Simulink-PS Converter4/RConn1 -- Planar Joint/LConn4
  Simulink-PS Converter3/RConn1 -- Planar Joint/LConn3
  Simulink-PS Converter2/RConn1 -- Planar Joint/LConn2
  Planar Joint/LConn1 -- Rigid Transform2/RConn1
  Simulink-PS Converter1/RConn1 -- Right Revolute Joint/LConn2
  Simulink-PS Converter/RConn1 -- Left Revolute Joint/LConn2
  Right Wheel/RConn1 -- Right Revolute Joint/RConn1
  Right Revolute Joint/LConn1 -- Rigid Transform1/RConn1
  Left Revolute Joint/LConn1 -- Rigid Transform/RConn1
  Left Wheel/RConn1 -- Left Revolute Joint/RConn1
  Rigid Transform/LConn1 -- R/RConn1 -- Base/RConn1 -- Rigid Transform1/LConn1 -- Planar Joint/RConn1
  Rigid Transform2/LConn1 -- G/RConn1

== system mobileRoboticsLib/Kinematic Models/Differential Drive/Differential Drive Forward Kinematics ==
  wheelSpd : Inport
  Demux : Demux  Outputs=2
  MATLAB Function : MATLAB Function  TreatAsAtomicUnit=on
  Mux : Mux  Inputs=2
  bodySpd : Outport
  wires:
  MATLAB Function/1(v) -> Mux/1  "v"
  MATLAB Function/2(w) -> Mux/2  "w"
  Mux/1 -> bodySpd/1
  wheelSpd/1 -> Demux/1
  Demux/1 -> MATLAB Function/1(wL)  "wL"
  Demux/2 -> MATLAB Function/2(wR)  "wR"

== system mobileRoboticsLib/Kinematic Models/Differential Drive/Differential Drive Inverse Kinematics ==
  vRef : Inport
  Demux : Demux  Outputs=2
  MATLAB Function : MATLAB Function  TreatAsAtomicUnit=on
  Mux : Mux  Inputs=2
  wheelSpd : Outport
  wires:
  Demux/2 -> MATLAB Function/2(w)  "w"
  Demux/1 -> MATLAB Function/1(v)  "v"
  vRef/1 -> Demux/1
  Mux/1 -> wheelSpd/1
  MATLAB Function/2(wR) -> Mux/2  "wR"
  MATLAB Function/1(wL) -> Mux/1  "wL"

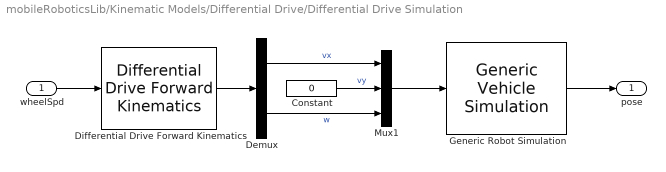
== system mobileRoboticsLib/Kinematic Models/Differential Drive/Differential Drive Simulation ==
  wheelSpd : Inport
  Constant : Constant  Value=0
  Demux : Demux  Outputs=2
  Differential Drive Forward Kinematics : $bdroot/Kinematic Models/Differential Drive/Differential Drive Forward Kinematics  wheelRadius=wheelRadius  wheelBase=wheelBase
  Generic Robot Simulation : $bdroot/Utilities/Generic Vehicle Simulation  OverrideUsingVariant=mode==2  initX=initX  initY=initY  initAngle=initAngle  Ts=Ts
  Mux1 : Mux  Inputs=3
  pose : Outport
  wires:
  Mux1/1 -> Generic Robot Simulation/1
  Demux/1 -> Mux1/1  "vx"
  Demux/2 -> Mux1/3  "w"
  Constant/1 -> Mux1/2  "vy"
  wheelSpd/1 -> Differential Drive Forward Kinematics/1
  Differential Drive Forward Kinematics/1 -> Demux/1
  Generic Robot Simulation/1 -> pose/1
